simulink model "test"  (R2018b)
settings: Solver=VariableStepAuto  StartTime=0.0  StopTime=10.0  RelTol=1e-3
settings Model: Creator=Leshi  LastModifiedBy=Leshi

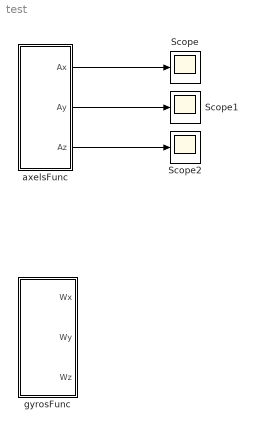
== system test ==
  Scope : Scope
  Scope1 : Scope
  Scope2 : Scope
  axelsFunc : MATLAB Function  TreatAsAtomicUnit=on
  gyrosFunc : MATLAB Function  TreatAsAtomicUnit=on
  wires:
  axelsFunc/1(Ax) -> Scope/1
  axelsFunc/2(Ay) -> Scope1/1
  axelsFunc/3(Az) -> Scope2/1

== matlab function test/gyrosFunc ==
  data: Wx output; Wy output; Wz output
% Give increment of anular vels
function [Wx, Wy, Wz] = Gyros()

Wx = awgn(0,10,'measured');
Wy = awgn(0,10,'measured');
Wz = awgn(0,10,'measured');

== matlab function test/axelsFunc ==
  data: Ax output; Ay output; Az output
% Give pure aceleration
function [Ax, Ay, Az] = Axels()

g = [0, 9.81, 0];

Q = quaternion(cos(30/57.3/2), 0, 0, sin(30/57.3/2));
[q0, q1, q2, q3] = parts(Q);
Q_ = quaternion(q0, -q1, -q2, -q3);

cQ = [q0^2 + q1^2 - q2^2 - q3^2, 2 * (q1 * q2 - q3 * q0),   2 * (q1 * q3 + q0 * q2);
     2 * (q1 * q2 + q0 * q3),   q0^2 - q1^2 + q2^2 - q3^2, 2 * (q2 * q3 - q0 * q1);
     2 * (q1 * q3 - q0 * q2),   2 * (q2 * q3 + q0 * q1),   q0^2 - q1^2 - q2^2 + q3^2];
 
[q0, q1, q2, q3] = parts(Q_);
 
cQ_ = [q0^2 + q1^2 - q2^2 - q3^2, 2 * (q1 * q2 - q3 * q0),   2 * (q1 * q3 + q0 * q2);
     2 * (q1 * q2 + q0 * q3),   q0^2 - q1^2 + q2^2 - q3^2, 2 * (q2 * q3 - q0 * q1);
     2 * (q1 * q3 - q0 * q2),   2 * (q2 * q3 + q0 * q1),   q0^2 - q1^2 - q2^2 + q3^2];
 
gCurrnet = g * cQ_;

% gCurrnet = [0, 1, 2];

Ax = gCurrnet(1);
Ay = gCurrnet(2);
Az = gCurrnet(3);

% Ax = normrnd(gCurrnet(1),0.03);
% Ay = normrnd(gCurrnet(2),0.03);
% Az = normrnd(gCurrnet(3),0.03);
